simulink model "PD_controller"  (R2022b)
settings: Solver=VariableStepAuto  StartTime=0.0  StopTime=10.0  RelTol=1e-3
libraries: simulink x1
settings Model: Creator=yasso  LastModifiedBy=yasso

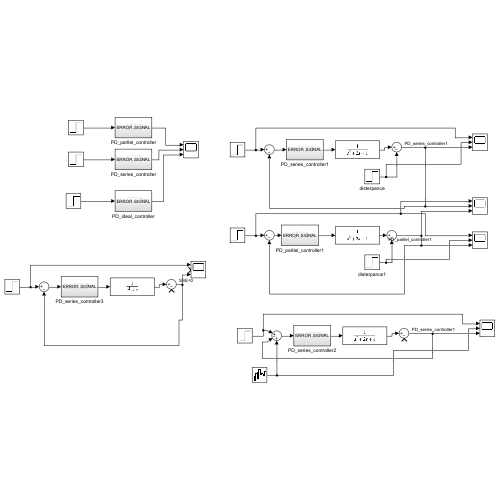
[thumbnail: Simulink's stored preview of the top-level diagram]
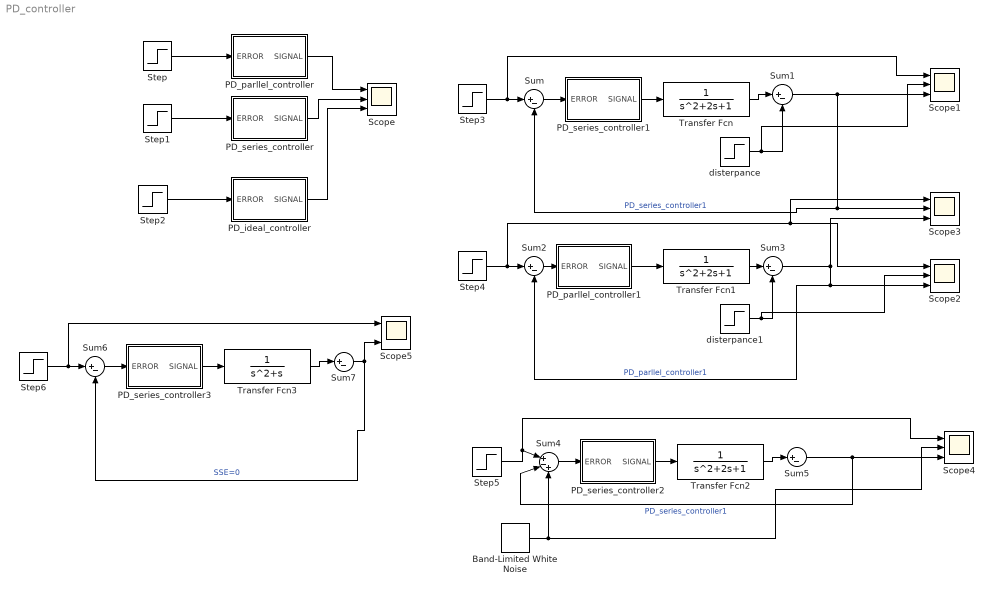
== system PD_controller ==
  Band-Limited White Noise : simulink/Sources/Band-Limited White Noise  Cov=[0.1]  Ts=0.1  seed=[23341]
  PD_ideal_controller : Subsystem
  PD_parllel_controller : Subsystem
  PD_parllel_controller1 : Subsystem
  PD_series_controller : Subsystem
  PD_series_controller1 : Subsystem
  PD_series_controller2 : Subsystem
  PD_series_controller3 : Subsystem
  Scope{,1..5} (6 alike) : Scope  NumInputPorts=3
  Step{,1..6} (7 alike) : Step  SampleTime=0
  Sum{,1..3,5..7} (7 alike) : Sum  Inputs=|+-
  Sum4 : Sum  Inputs=|+-+
  Transfer Fcn : TransferFcn
  Transfer Fcn1 : TransferFcn
  Transfer Fcn2 : TransferFcn
  Transfer Fcn3 : TransferFcn  Denominator=[1 1 0]
  disterpance : Step  Time=4  After=0.4  SampleTime=0
  disterpance1 : Step  Time=4  After=0.4  SampleTime=0
  wires:
  Sum/1 -> PD_series_controller1/1(ERROR)
  Step4/1 -> Sum2/1, Scope2/1, Scope3/1
  PD_parllel_controller/1(SIGNAL) -> Scope/1
  PD_ideal_controller/1(SIGNAL) -> Scope/3
  Sum2/1 -> PD_parllel_controller1/1(ERROR)
  Step2/1 -> PD_ideal_controller/1(ERROR)
  disterpance1/1 -> Sum3/2, Scope2/2
  Sum3/1 -> Scope3/3, Sum2/2, Scope2/3  "PD_parllel_controller1"
  Transfer Fcn1/1 -> Sum3/1
  disterpance/1 -> Scope1/2, Sum1/2
  Sum1/1 -> Sum/2, Scope3/2, Scope1/3  "PD_series_controller1"
  PD_series_controller/1(SIGNAL) -> Scope/2
  PD_series_controller1/1(SIGNAL) -> Transfer Fcn/1
  Step3/1 -> Scope1/1, Sum/1
  Step1/1 -> PD_series_controller/1(ERROR)
  PD_parllel_controller1/1(SIGNAL) -> Transfer Fcn1/1
  Step/1 -> PD_parllel_controller/1(ERROR)
  Transfer Fcn/1 -> Sum1/1
  Transfer Fcn2/1 -> Sum5/1
  Step5/1 -> Sum4/1, Scope4/1
  PD_series_controller2/1(SIGNAL) -> Transfer Fcn2/1
  Sum5/1 -> Scope4/3, Sum4/2  "PD_series_controller1"
  Band-Limited White Noise/1 -> Scope4/2, Sum4/3
  Sum4/1 -> PD_series_controller2/1(ERROR)
  Transfer Fcn3/1 -> Sum7/1
  Step6/1 -> Sum6/1, Scope5/1
  PD_series_controller3/1(SIGNAL) -> Transfer Fcn3/1
  Sum7/1 -> Scope5/3, Sum6/2  "SSE=0"
  Sum6/1 -> PD_series_controller3/1(ERROR)

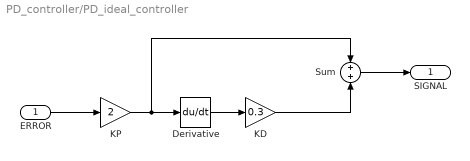
== system PD_controller/PD_ideal_controller ==
  ERROR : Inport
  Derivative : Derivative
  KD : Gain  Gain=0.3
  KP : Gain  Gain=2
  Sum : Sum  Inputs=+|+
  SIGNAL : Outport
  wires:
  KP/1 -> Derivative/1, Sum/1
  KD/1 -> Sum/2
  ERROR/1 -> KP/1
  Derivative/1 -> KD/1
  Sum/1 -> SIGNAL/1

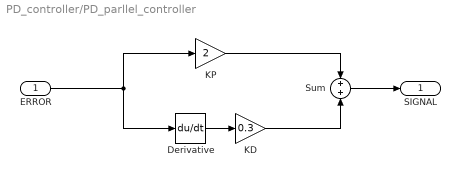
== system PD_controller/PD_parllel_controller ==
  ERROR : Inport
  Derivative : Derivative
  KD : Gain  Gain=0.3
  KP : Gain  Gain=2
  Sum : Sum  Inputs=+|+
  SIGNAL : Outport
  wires:
  KD/1 -> Sum/2
  ERROR/1 -> Derivative/1, KP/1
  KP/1 -> Sum/1
  Derivative/1 -> KD/1
  Sum/1 -> SIGNAL/1

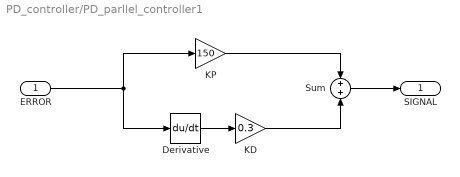
== system PD_controller/PD_parllel_controller1 ==
  ERROR : Inport
  Derivative : Derivative
  KD : Gain  Gain=0.3
  KP : Gain  Gain=150
  Sum : Sum  Inputs=+|+
  SIGNAL : Outport
  wires:
  Sum/1 -> SIGNAL/1
  Derivative/1 -> KD/1
  KP/1 -> Sum/1
  ERROR/1 -> Derivative/1, KP/1
  KD/1 -> Sum/2

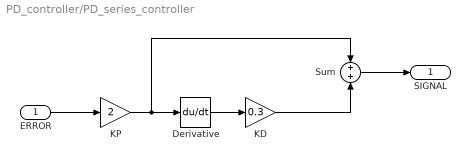
== system PD_controller/PD_series_controller ==
  ERROR : Inport
  Derivative : Derivative
  KD : Gain  Gain=0.3
  KP : Gain  Gain=2
  Sum : Sum  Inputs=+|+
  SIGNAL : Outport
  wires:
  Sum/1 -> SIGNAL/1
  Derivative/1 -> KD/1
  ERROR/1 -> KP/1
  KD/1 -> Sum/2
  KP/1 -> Derivative/1, Sum/1

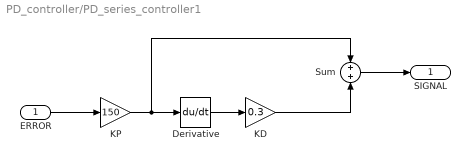
== system PD_controller/PD_series_controller1 ==
  ERROR : Inport
  Derivative : Derivative
  KD : Gain  Gain=0.3
  KP : Gain  Gain=150
  Sum : Sum  Inputs=+|+
  SIGNAL : Outport
  wires:
  KP/1 -> Derivative/1, Sum/1
  KD/1 -> Sum/2
  ERROR/1 -> KP/1
  Derivative/1 -> KD/1
  Sum/1 -> SIGNAL/1

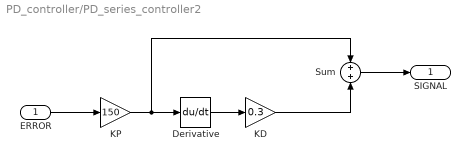
== system PD_controller/PD_series_controller2 ==
  ERROR : Inport
  Derivative : Derivative
  KD : Gain  Gain=0.3
  KP : Gain  Gain=150
  Sum : Sum  Inputs=+|+
  SIGNAL : Outport
  wires:
  Sum/1 -> SIGNAL/1
  Derivative/1 -> KD/1
  ERROR/1 -> KP/1
  KD/1 -> Sum/2
  KP/1 -> Sum/1, Derivative/1

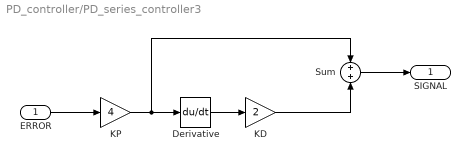
== system PD_controller/PD_series_controller3 ==
  ERROR : Inport
  Derivative : Derivative
  KD : Gain  Gain=2
  KP : Gain  Gain=4
  Sum : Sum  Inputs=+|+
  SIGNAL : Outport
  wires:
  Sum/1 -> SIGNAL/1
  Derivative/1 -> KD/1
  ERROR/1 -> KP/1
  KD/1 -> Sum/2
  KP/1 -> Sum/1, Derivative/1
